simulink model "simpleEqnBased"  (R2018a)
settings: Solver=VariableStepAuto  StartTime=0.0  StopTime=10.0  RelTol=1e-3
undefined symbols (not defined in the file): veh
settings Model: Creator=carca  LastModifiedBy=carca

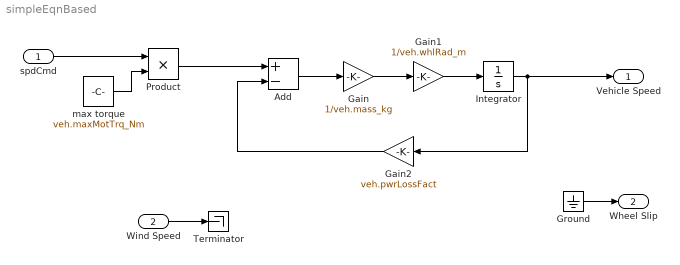
== system simpleEqnBased ==
  spdCmd : Inport
  Wind Speed : Inport  Port=2
  Add : Sum  Inputs=+-
  Gain : Gain  Gain=1/veh.mass_kg
  Gain1 : Gain  Gain=1/veh.whlRad_m
  Gain2 : Gain  Gain=veh.pwrLossFact
  Ground : Ground
  Integrator : Integrator
  Product : Product
  Terminator : Terminator
  max torque : Constant  Value=veh.maxMotTrq_Nm
  Vehicle Speed : Outport
  Wheel Slip : Outport  Port=2
  wires:
  Add/1 -> Gain/1
  Gain/1 -> Gain1/1
  Gain1/1 -> Integrator/1
  Integrator/1 -> Vehicle Speed/1, Gain2/1
  Gain2/1 -> Add/2
  Ground/1 -> Wheel Slip/1
  Wind Speed/1 -> Terminator/1
  spdCmd/1 -> Product/1
  Product/1 -> Add/1
  max torque/1 -> Product/2
